simulink model "PE2_Ex11R2017a"  (R2017a)
settings: Solver=VariableStepAuto  StartTime=0.0  StopTime=0.08  RelTol=1e-3
libraries: powerlib x15
settings Model: Creator=ASUS  LastModifiedBy=ASUS
settings DataIOCC: ReturnWorkspaceOutputs=on
settings SFSimCC: SimUseLocalCustomCode=on
settings RTWCC: RTWUseLocalCustomCode=on

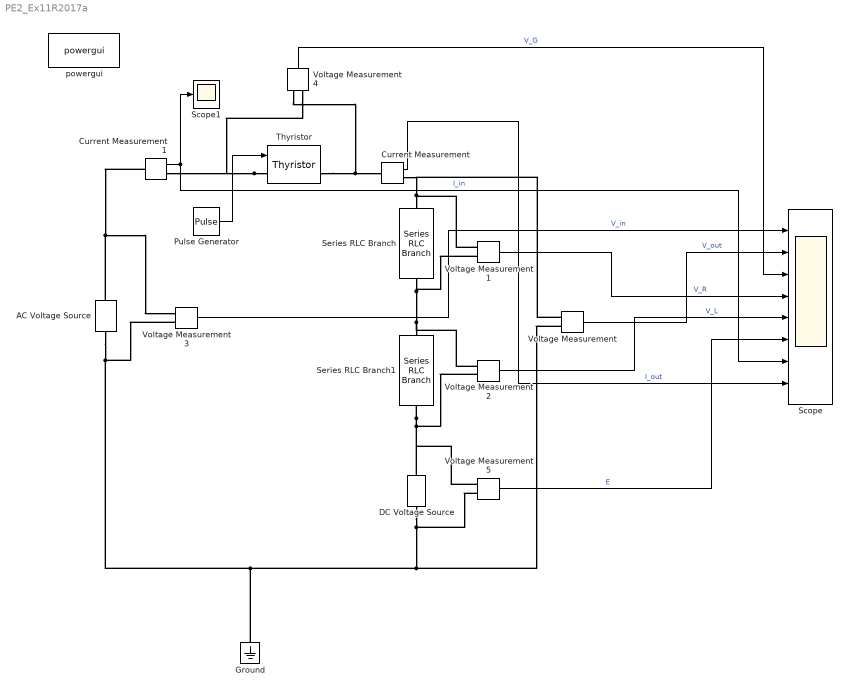
== system PE2_Ex11R2017a ==
  AC Voltage Source : powerlib/Electrical Sources/AC Voltage Source  Amplitude=339.41  Phase=0  Frequency=60  SampleTime=0  Measurements=None  BusType=swing  Pref=10e3  Qref=0  Qmin=-inf  Qmax=+inf
  Current Measurement : powerlib/Measurements/Current Measurement  PhasorSimulation=off  OutputType=Complex  PSBequivalent=0
  Current Measurement1 : powerlib/Measurements/Current Measurement  PhasorSimulation=off  OutputType=Complex  PSBequivalent=0
  DC Voltage Source : powerlib/Electrical Sources/DC Voltage Source  Amplitude=96  Measurements=None
  Ground : powerlib/Elements/Ground  LConnTagsString=a
  Pulse Generator : DiscretePulseGenerator  PulseType=Time based  Period=1/60  PulseWidth=50  PhaseDelay=0.00277866
  Scope : Scope  NumInputPorts=8
  Scope1 : Scope
  Series RLC Branch : powerlib/Elements/Series RLC Branch  LConnTagsString=__new0  RConnTagsString=__new0  BranchType=R  Resistance=100  Inductance=1e-3  SetiL0=off  InitialCurrent=0  Capacitance=1e-6  Setx0=off  InitialVoltage=0  Measurements=None
  Series RLC Branch1 : powerlib/Elements/Series RLC Branch  LConnTagsString=__new0  RConnTagsString=__new0  BranchType=L  Resistance=1  Inductance=150e-3  SetiL0=off  InitialCurrent=0  Capacitance=1e-6  Setx0=off  InitialVoltage=0  Measurements=None
  Thyristor : powerlib/Power Electronics/Thyristor  Ron=0.001  Lon=0  Vf=0.6  IC=0  Rs=0  Cs=0  Measurements=on
  Voltage Measurement{,1..5} (6 alike) : powerlib/Measurements/Voltage Measurement  PhasorSimulation=off  OutputType=Complex  PSBequivalent=0
  powergui : powerlib/powergui  Priority=1  SimulationMode=Continuous  SampleTime=50e-6  frequency=60  Iterations=50  frequencyindice=60  Pbase=100e6  ErrMax=1e-4  UnitsV=kV  UnitsW=MW  buscounter=0  FunctionMessages=off  echomessages=off  EnableUseOfTLC=off  CurrentSourceSwitches=off  DisableSnubberDevices=off  DisableRonSwitches=off  DisableVfSwitches=off  DisplayEquations=off  AutomaticDiscreteSolvers=off  SolverType=Tustin/Backward Euler (TBE)  Interpol=off  ExternalGateDelay=off  methode=off  Ts=100  x0status=blocks  SPID=on  SwTol=0  HookPort=off  NonlinearTolerance=1e-4  nMaxIteration=100  ContinueOnMaxIteration=off  RestoreLinks=warning  ResistiveCurrentMeasurement=off  Frange=[0:2:500]  Ylog=off  Xlog=on  ShowGrid=off  save=off  variable=ZData  structure=0  ZoomFFT=off  StartTime=0.0  cycles=1  DisplayStyle=1  fundamental=60  FreqAxis=off  MaxFrequency=1000  frequencyindicesteady=1  RmsSteady=1  display=off
  wires:
  Current Measurement/1 -> Scope/8  "I_out"
  Voltage Measurement4/1 -> Scope/3  "V_G"
  Voltage Measurement1/1 -> Scope/4  "V_R"
  Current Measurement1/1 -> Scope1/1, Scope/7  "I_in"
  Voltage Measurement/1 -> Scope/2  "V_out"
  Voltage Measurement2/1 -> Scope/5  "V_L"
  Pulse Generator/1 -> Thyristor/1
  Voltage Measurement3/1 -> Scope/1  "V_in"
  Voltage Measurement5/1 -> Scope/6  "E"
  connections:
  Thyristor/RConn1 -- Voltage Measurement4/LConn1 -- Current Measurement/LConn1
  Series RLC Branch/LConn1 -- Voltage Measurement1/LConn1 -- Voltage Measurement/LConn1 -- Current Measurement/RConn1
  Series RLC Branch/RConn1 -- Voltage Measurement1/LConn2 -- Voltage Measurement2/LConn1 -- Series RLC Branch1/LConn1
  Thyristor/LConn1 -- Current Measurement1/RConn1 -- Voltage Measurement4/LConn2
  DC Voltage Source/LConn1 -- Voltage Measurement/LConn2 -- Ground/LConn1 -- Voltage Measurement3/LConn2 -- AC Voltage Source/LConn1 -- Voltage Measurement5/LConn2
  Current Measurement1/LConn1 -- Voltage Measurement3/LConn1 -- AC Voltage Source/RConn1
  Series RLC Branch1/RConn1 -- Voltage Measurement5/LConn1 -- DC Voltage Source/RConn1 -- Voltage Measurement2/LConn2
